simulink model "Motor_Pos_Ctrl"  (R2020a)
settings: Solver=ode15s  StartTime=0.0  StopTime=0.2  RelTol=1e-3
undefined symbols (not defined in the file): b, J, K, L, R
settings Model: Creator=NIKITA  LastModifiedBy=NIKITA

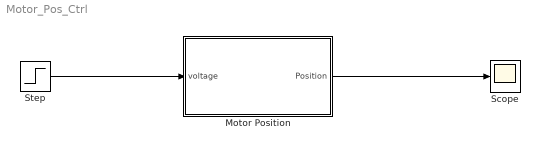
== system Motor_Pos_Ctrl ==
  Motor Position : Subsystem
  Scope : Scope
  Step : Step  Time=0  SampleTime=0
  wires:
  Step/1 -> Motor Position/1(voltage)
  Motor Position/1(Position) -> Scope/1

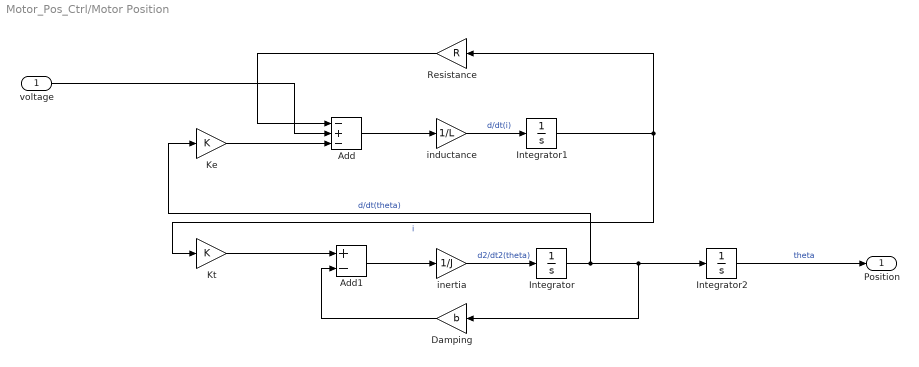
== system Motor_Pos_Ctrl/Motor Position ==
  voltage : Inport
  Add : Sum  Inputs=-+-
  Add1 : Sum  Inputs=+-
  Damping : Gain  Gain=b
  Integrator : Integrator
  Integrator1 : Integrator
  Integrator2 : Integrator
  Ke : Gain  Gain=K
  Kt : Gain  Gain=K
  Resistance : Gain  Gain=R
  inductance : Gain  Gain=1/L
  inertia : Gain  Gain=1/J
  Position : Outport
  wires:
  Kt/1 -> Add1/1
  Resistance/1 -> Add/1
  Integrator/1 -> Ke/1, Integrator2/1, Damping/1  "d/dt(theta)"
  inductance/1 -> Integrator1/1  "d/dt(i)"
  Damping/1 -> Add1/2
  inertia/1 -> Integrator/1  "d2/dt2(theta)"
  Integrator1/1 -> Resistance/1, Kt/1  "i"
  Add/1 -> inductance/1
  Ke/1 -> Add/3
  Add1/1 -> inertia/1
  Integrator2/1 -> Position/1  "theta"
  voltage/1 -> Add/2
